simulink model "GyroscopeHinfinityController"  (Simulink 8.5)
settings: Solver=ode1  StartTime=0.0  StopTime=inf  FixedStep=0.002  MaxStep=10  RelTol=1e-3  AbsTol=1e-3
values from neighbouring files (symbols this model uses):
  ac = contr(1:n,1:n)    [HinfinityController.m]
  bc = contr(1:n,n+1)    [HinfinityController.m]
  cc = contr(n+1,1:n)    [HinfinityController.m]
  dc = contr(n+1,n+1)    [HinfinityController.m]
undefined symbols (not defined in the file or in its folder): HIL
libraries: quarc_library x4, simulink_extras x2
settings Model: Creator=MLevis  LastModifiedBy=gyroscope  SimulationMode=external  ExtModeTrigDuration=10000
settings SolverCC: PositivePriorityOrder=on
settings DataIOCC: LimitDataPoints=off  SaveOutput=off  SaveTime=off  SignalLoggingName=sigsOut
settings OptimizationCC: BlockReduction=off  BooleanDataType=off  OptimizeBlockIOStorage=off  BufferReuse=off  GlobalBufferReuse=off  ExpressionFolding=off  LocalBlockOutputs=off  InitFltsAndDblsToZero=on
settings DebuggingCC: SaveWithParameterizedLinksMsg=none  SignalResolutionControl=TryResolveAllWithWarning  MultiTaskDSMMsg=warning  MultiTaskCondExecSysMsg=none  FcnCallInpInsideContextMsg=UseLocalSettings
settings HardwareCC: TargetHWDeviceType=32-bit Generic
settings RTWCC: SystemTargetFile=quarc_win64.tlc  TemplateMakefile=quarc_default_tmf  Description=QUARC Win64 Target
settings STFCustomTargetCC: TargetPreCompLibLocation=C:\PROGRA~3\QUARC\lib\2015a\win64\release  ConcurrentExecutionCompliant=on  GeneratePreprocessorConditionals=Disable all  CPPClassGenCompliant=on  SystemTargetFile=quarc_win64.tlc
settings GRTTargetCC: TargetPreCompLibLocation=C:\PROGRA~3\QUARC\lib\2015a\win64\release  ParMdlRefBuildCompliant=off  CompOptLevelCompliant=off  MatFileLogging=off  ExtMode=on  ExtModeMexFile=quarc_comm

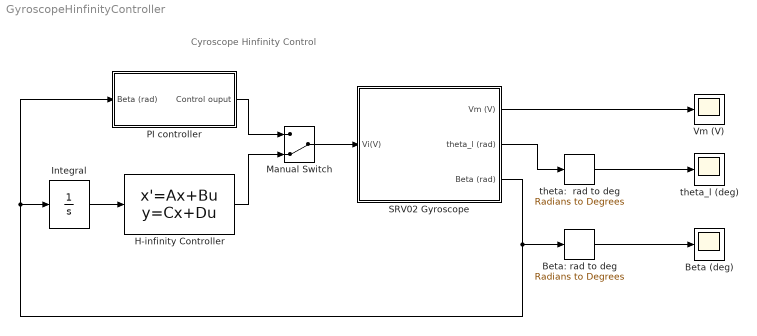
== system GyroscopeHinfinityController ==
  note: Cyroscope Hinfinity Control
  Beta (deg) : Scope
      settings: TimeRange=10  YMin=-17.5  YMax=17.5  SaveName=data_alpha
  Beta: rad to deg : simulink_extras/Transformations/Radians to Degrees
  H-infinity Controller : StateSpace  A=ac  B=bc  C=cc  D=dc  X0=0
  Integral : Integrator  LimitOutput=on  UpperSaturationLimit=5*pi/180  LowerSaturationLimit=-5*pi/180
  Manual Switch : ManualSwitch  CurrentSetting=0
  PI controller : Subsystem
  SRV02 Gyroscope : Subsystem
  Vm (V) : Scope
      settings: TickLabels=on  TimeRange=10  YMin=-15  YMax=15  SaveName=data_vm
  theta:  rad to deg : simulink_extras/Transformations/Radians to Degrees
  theta_l (deg) : Scope
      settings: TimeRange=10  YMin=-10  YMax=7.5  SaveName=data_theta
  wires:
  SRV02 Gyroscope/1(Vm (V)) -> Vm (V)/1
  SRV02 Gyroscope/2(theta_l (rad)) -> theta:  rad to deg/1
  Manual Switch/1 -> SRV02 Gyroscope/1(Vi(V))
  PI controller/1("Control ouput ") -> Manual Switch/1
  Beta: rad to deg/1 -> Beta (deg)/1
  theta:  rad to deg/1 -> theta_l (deg)/1
  H-infinity Controller/1 -> Manual Switch/2
  SRV02 Gyroscope/3(Beta (rad)) -> Integral/1, PI controller/1(Beta (rad)), Beta: rad to deg/1
  Integral/1 -> H-infinity Controller/1

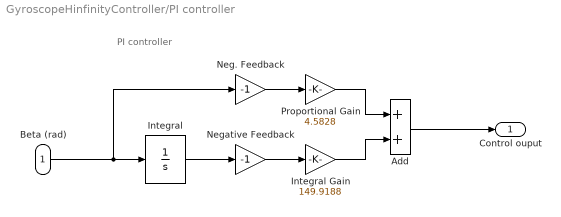
== system GyroscopeHinfinityController/PI controller ==
  note: PI controller
  Beta (rad) : Inport
  Add : Sum
  Integral : Integrator  LimitOutput=on  UpperSaturationLimit=5*pi/180  LowerSaturationLimit=-5*pi/180
  Integral Gain : Gain  Gain=149.9188
  Neg. Feedback : Gain  Gain=-1
  Negative Feedback : Gain  Gain=-1
  Proportional Gain : Gain  Gain=4.5828
  "Control ouput " : Outport
  wires:
  Beta (rad)/1 -> Neg. Feedback/1, Integral/1
  Add/1 -> "Control ouput "/1
  Integral/1 -> Negative Feedback/1
  Neg. Feedback/1 -> Proportional Gain/1
  Proportional Gain/1 -> Add/1
  Integral Gain/1 -> Add/2
  Negative Feedback/1 -> Integral Gain/1

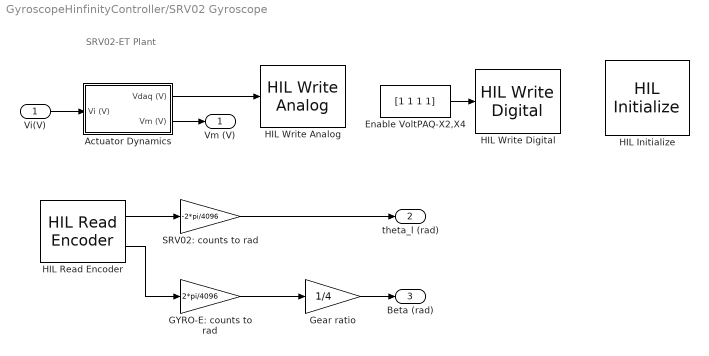
== system GyroscopeHinfinityController/SRV02 Gyroscope ==
  note: SRV02-ET Plant
  Vi(V) : Inport
  Actuator Dynamics : Subsystem
  Enable VoltPAQ-X2,X4 : Constant  Value=[1 1 1 1]
  GYRO-E: counts to rad : Gain  Gain=2*pi/4096
  Gear ratio : Gain  Gain=1/4  SaturateOnIntegerOverflow=on  OutDataTypeStr=Inherit: Same as input  ParamDataTypeStr=Inherit: Same as input
  HIL Initialize : quarc_library/Data Acquisition/Generic/Configuration/HIL Initialize  object_name=HIL-1  board_type=q2_usb  board_number=0  board_options=d0=digital;d1=digital;led=auto;update_rate=normal  exclusive=off  active=off  hardware_clocks=[0:2]  clock_modes=[]  initial_clock_frequencies=[]  set_clock_params_at_start=off  set_clock_params_at_switch_in=off  set_clock_frequencies_at_start=off  set_clock_frequencies_at_switch_in=off  analog_input_channels=[0:1]  analog_input_maximums=10  analog_input_minimums=-10  set_analog_input_params_at_start=on  set_analog_input_params_at_switch_in=off  analog_output_channels=[0:1]  analog_output_maximums=10  analog_output_minimums=-10  initial_analog_outputs=[0]  final_analog_outputs=[0]  watchdog_analog_outputs=0  set_analog_output_params_at_start=on  set_analog_output_params_at_switch_in=off  set_analog_outputs_at_start=on  set_analog_outputs_at_switch_in=off  set_analog_outputs_at_terminate=on  set_analog_outputs_at_switch_out=off  set_analog_outputs_on_watchdog=off  digital_input_channels=[]  digital_output_channels=[0:7]  digital_output_configuration=[]  initial_digital_outputs=[0]  final_digital_outputs=[0]  watchdog_digital_outputs=[0]  set_digital_output_params_at_start=off  set_digital_output_params_at_switch_in=off  set_digital_outputs_at_start=on  set_digital_outputs_at_switch_in=off  set_digital_outputs_at_terminate=on  set_digital_outputs_at_switch_out=off  set_digital_outputs_on_watchdog=off  encoder_channels=[0:1]  quadrature=[4]  encoder_filter_frequency=[]  initial_encoder_counts=[0]  set_encoder_params_at_start=on  set_encoder_params_at_switch_in=off  set_encoder_counts_at_start=on  set_encoder_counts_at_switch_in=off  pwm_channels=[]  pwm_modes=[0]  pwm_frequency=1/0.020  pwm_configuration=[]  pwm_alignment=[]  pwm_polarity=[]  pwm_leading_deadband=[]  pwm_trailing_deadband=[]  initial_pwm_outputs=[0]  final_pwm_outputs=[0]  watchdog_pwm_outputs=[0]  set_pwm_params_at_start=on  set_pwm_params_at_switch_in=off  set_pwm_outputs_at_start=on  set_pwm_outputs_at_switch_in=off  set_pwm_outputs_at_terminate=on  set_pwm_outputs_at_switch_out=off  set_pwm_outputs_on_watchdog=off  other_output_channels=[]  initial_other_outputs=[]  final_other_outputs=[]  watchdog_other_outputs=[]  set_other_outputs_at_start=off  set_other_outputs_at_switch_in=off  set_other_outputs_at_terminate=off  set_other_outputs_at_switch_out=off  set_other_outputs_on_watchdog=off
  HIL Read Encoder : quarc_library/Data Acquisition/Generic/Immediate I//O/HIL Read Encoder  Tag=unassigned  object_name=HIL-1  channels=[0:1]  sample_time=qc_get_step_size  active=on  vector_output=off  data_type_mode=Inherit via back propagation  data_type=double
  HIL Write Analog : quarc_library/Data Acquisition/Generic/Immediate I//O/HIL Write Analog  Tag=unassigned  object_name=HIL-1  channels=0  sample_time=-1  active=off  vector_input=off
  HIL Write Digital : quarc_library/Data Acquisition/Generic/Immediate I//O/HIL Write Digital  object_name=HIL-1  channels=[0:3]  sample_time=-1  active=off  vector_input=on
  SRV02: counts to rad : Gain  Gain=-2*pi/4096
  Vm (V) : Outport  InitialOutput=0
  theta_l (rad) : Outport  Port=2  InitialOutput=0
  Beta (rad) : Outport  Port=3  InitialOutput=0
  wires:
  Vi(V)/1 -> Actuator Dynamics/1(Vi (V))
  Actuator Dynamics/1(Vdaq (V)) -> HIL Write Analog/1
  Actuator Dynamics/2(Vm (V)) -> Vm (V)/1
  HIL Read Encoder/1 -> SRV02: counts to rad/1
  SRV02: counts to rad/1 -> theta_l (rad)/1
  GYRO-E: counts to rad/1 -> Gear ratio/1
  Gear ratio/1 -> Beta (rad)/1
  Enable VoltPAQ-X2,X4/1 -> HIL Write Digital/1
  HIL Read Encoder/2 -> GYRO-E: counts to rad/1

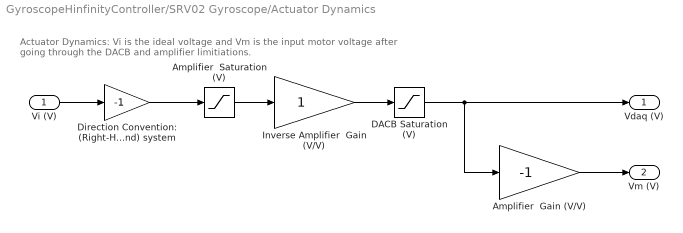
== system GyroscopeHinfinityController/SRV02 Gyroscope/Actuator Dynamics ==
  note: Actuator Dynamics: Vi is the ideal voltage and Vm is the
      | input motor voltage after going through the DACB and amplifier limitiations.
  Vi (V) : Inport
  Amplifier  Gain (V/V) : Gain  Gain=-1
  Amplifier  Saturation (V) : Saturate  UpperLimit=10  LowerLimit=-10
  DACB Saturation (V) : Saturate  UpperLimit=10  LowerLimit=-10
  Direction Convention: (Right-Hand) system : Gain  Gain=-1  SaturateOnIntegerOverflow=on  OutDataTypeStr=Inherit: Same as input  ParamDataTypeStr=Inherit: Same as input
  Inverse Amplifier  Gain (V/V) : Gain
  Vdaq (V) : Outport
  Vm (V) : Outport  Port=2
  wires:
  Vi (V)/1 -> Direction Convention: (Right-Hand) system/1
  Amplifier  Saturation (V)/1 -> Inverse Amplifier  Gain (V/V)/1
  Inverse Amplifier  Gain (V/V)/1 -> DACB Saturation (V)/1
  DACB Saturation (V)/1 -> Amplifier  Gain (V/V)/1, Vdaq (V)/1
  Amplifier  Gain (V/V)/1 -> Vm (V)/1
  Direction Convention: (Right-Hand) system/1 -> Amplifier  Saturation (V)/1
